simulink model "fixed_point_iteration"  (R2021a)
settings: Solver=FixedStepDiscrete  StartTime=0.0  StopTime=inf  FixedStep=1  RelTol=1e-3
libraries: simulink x1
settings Model: Creator=manur  LastModifiedBy=manur

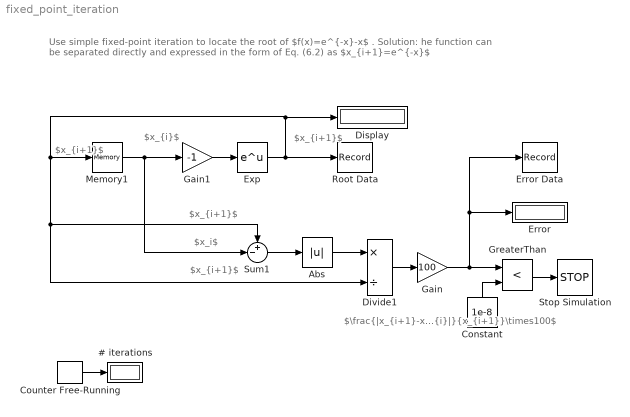
== system fixed_point_iteration ==
  note: $x_{i+1}$
  note: Use simple fixed-point iteration to locate the root of $f(x)=e^{-x}-x$ .
      |
      | Solution: he function can be separated directly and expressed in the form of Eq. (6.2) as $x_{i+1}=e^{-x}$
  note: $x_{i+1}$
  note: $\frac{|x_{i+1}-x_{i}|}{x_{i+1}}\times100$
  note: $x_{i+1}$
  note: $x_i$
  note: $x_{i+1}$
  note: $x_{i}$
  # iterations : Display
  Abs : Abs
  Constant : Constant  Value=1e-8
  Counter Free-Running : simulink/Sources/Counter Free-Running  NumBits=16  tsamp=-1
  Display : Display
  Divide1 : Product  Inputs=*/
  Error : Display
  Error Data : Record  FileSettingsInternal="{\"entries\":[{\"content\":{\"excelSettings\":{\"content\":{},\"type\":\"Streamout.ExcelSettings\"}},\"type\":\"Streamout.FileSettingStorage\",\"uuid\":\"f0071751-1568-4622-84f8-59859e537be1\"}],\"packageUris\":[\"http://schema.mathworks.com/mf0/streamout_blocks/R2020a\"],\"version\":\"1.0\"}"  SignalsInternal="{\"entries\":[{\"content\":{\"signals\":[{\"content\":{\"blockPath\":[\"fixed_point_iteration/Error Data\"],\"channel\":[],\"dimensions\":[1],\"domain\":\"fixed_point_iteration/error data\",\"lineColor\":\"#fe330a\",\"plots\":[1],\"port\":1,\"sid\":[],\"signalID\":57,\"signalName\":\"Gain\"},\"type\":\"RecordBlkView.Signal\",\"uuid\":\"8546414e-9ac8-4ea8-800e-f1da5b08f58d\"}]},\"type\":\"RecordBlkView.InputSignals\",\"uuid\":\"43f4dbdb-9b36-4694-8889-c6ca150c8ad5\"}],\"packageUris\":[\"http://schema.mathworks.com/mf0/streamout_blocks/R2020a\"],\"version\":\"1.0\"}"  VisualizationBindings="{\"sparklinesplugin\":{\"info\":[{\"bindingParametersList\":[],\"subplotID\":1}]}}"
  Exp : Math  SignedPower=on  SaturateOnIntegerOverflow=on
  Gain : Gain  Gain=100
  Gain1 : Gain  Gain=-1
  GreaterThan : RelationalOperator  Operator=<  OutDataTypeStr=boolean  RndMeth=Simplest
  Memory1 : Memory
  Root Data : Record  FileSettingsInternal="{\"entries\":[{\"content\":{\"excelSettings\":{\"content\":{},\"type\":\"Streamout.ExcelSettings\"}},\"type\":\"Streamout.FileSettingStorage\",\"uuid\":\"2d0c44c1-073e-486d-9f59-da843e532316\"}],\"packageUris\":[\"http://schema.mathworks.com/mf0/streamout_blocks/R2020a\"],\"version\":\"1.0\"}"  SignalsInternal="{\"entries\":[{\"content\":{\"signals\":[{\"content\":{\"blockPath\":[\"fixed_point_iteration/Root Data\"],\"channel\":[],\"dimensions\":[1],\"domain\":\"fixed_point_iteration/root data\",\"lineColor\":\"#b746ff\",\"plots\":[1],\"port\":1,\"sid\":[],\"signalID\":52,\"signalName\":\"Exp\"},\"type\":\"RecordBlkView.Signal\",\"uuid\":\"26e08dc8-8eea-4405-9480-7d72ecb15baf\"}]},\"type\":\"RecordBlkView.InputSignals\",\"uuid\":\"88b60a22-ac91-400d-9303-4b074ed4c122\"}],\"packageUris\":[\"http://schema.mathworks.com/mf0/streamout_blocks/R2020a\"],\"version\":\"1.0\"}"  VisualizationBindings="{\"sparklinesplugin\":{\"info\":[{\"bindingParametersList\":[],\"subplotID\":1}]}}"
  Stop Simulation : Stop
  Sum1 : Sum  Inputs=+-|
  wires:
  Exp/1 -> Divide1/2, Sum1/1, Memory1/1, Display/1, Root Data/1
  Sum1/1 -> Abs/1
  Divide1/1 -> Gain/1
  Abs/1 -> Divide1/1
  Constant/1 -> GreaterThan/2
  GreaterThan/1 -> Stop Simulation/1
  Gain/1 -> GreaterThan/1, Error/1, Error Data/1
  Counter Free-Running/1 -> # iterations/1
  Memory1/1 -> Sum1/2, Gain1/1
  Gain1/1 -> Exp/1
